simulink model "RealModel"  (R2016a)
settings: Solver=VariableStepAuto  StartTime=0.0  StopTime=10.0  RelTol=1e-3
undefined symbols (not defined in the file or in its folder): K
(part 1 of 7)
settings Model: Creator=Michael  LastModifiedBy=Michael

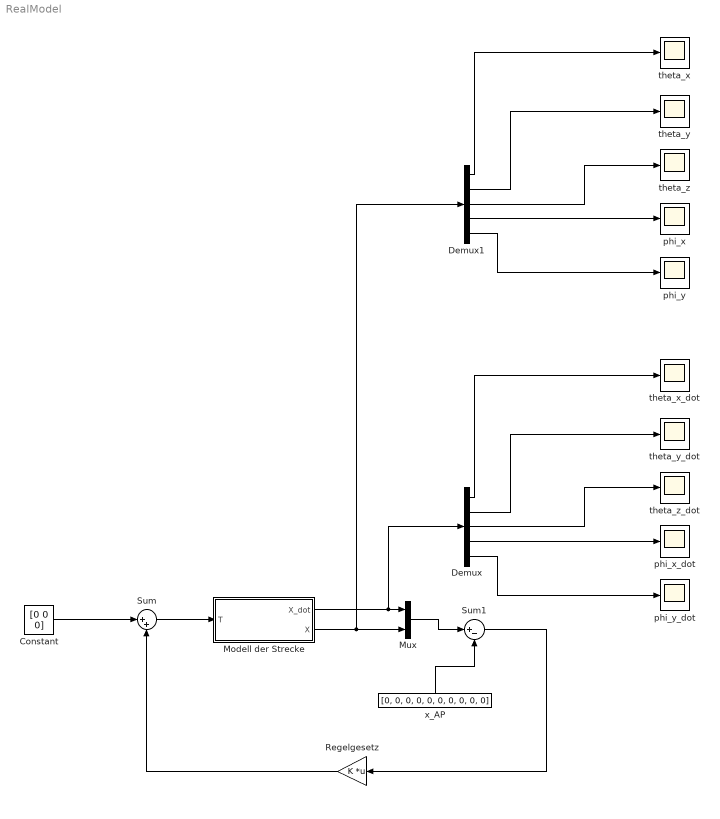
== system RealModel ==
  Constant : Constant  Value=[0 0 0]
  Demux : Demux  Outputs=5
  Demux1 : Demux  Outputs=5
  Modell der Strecke : Subsystem
  Mux : Mux  Inputs=2
  Regelgesetz : Gain  Gain=K  Multiplication=Matrix(K*u)
  Sum : Sum  Inputs=|++
  Sum1 : Sum  Inputs=|+-
  phi_x : Scope
  phi_x_dot : Scope
  phi_y : Scope
  phi_y_dot : Scope
  theta_x : Scope
  theta_x_dot : Scope
  theta_y : Scope
  theta_y_dot : Scope
  theta_z : Scope
  theta_z_dot : Scope
  x_AP : Constant  Value=[0, 0, 0, 0, 0, 0, 0, 0, 0, 0]  VectorParams1D=off
  wires:
  Sum/1 -> Modell der Strecke/1(T)
  Constant/1 -> Sum/1
  x_AP/1 -> Sum1/2
  Sum1/1 -> Regelgesetz/1
  Regelgesetz/1 -> Sum/2
  Demux/1 -> theta_x_dot/1
  Demux/2 -> theta_y_dot/1
  Demux/3 -> theta_z_dot/1
  Demux/4 -> phi_x_dot/1
  Demux/5 -> phi_y_dot/1
  Modell der Strecke/1(X_dot) -> Demux/1, Mux/1
  Modell der Strecke/2(X) -> Demux1/1, Mux/2
  Mux/1 -> Sum1/1
  Demux1/1 -> theta_x/1
  Demux1/2 -> theta_y/1
  Demux1/3 -> theta_z/1
  Demux1/4 -> phi_x/1
  Demux1/5 -> phi_y/1

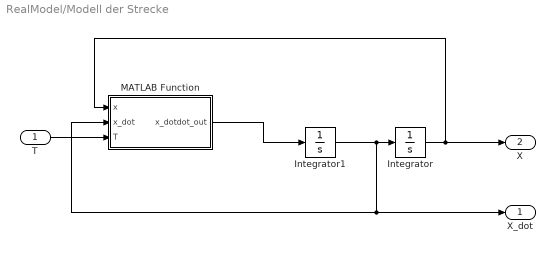
== system RealModel/Modell der Strecke ==
  T : Inport
  Integrator : Integrator  InitialCondition=[0 pi/32 0 0 0]
  Integrator1 : Integrator  InitialCondition=[0 0 0 0 0]
  MATLAB Function : MATLAB Function  TreatAsAtomicUnit=on
  X_dot : Outport
  X : Outport  Port=2
  wires:
  T/1 -> MATLAB Function/3(T)
  MATLAB Function/1(x_dotdot_out) -> Integrator1/1
  Integrator/1 -> MATLAB Function/1(x), X/1
  Integrator1/1 -> X_dot/1, MATLAB Function/2(x_dot), Integrator/1
